simulink model "problem2"  (R2020b)
settings: Solver=VariableStepAuto  StartTime=0.0  StopTime=10.0  RelTol=1e-3
values from neighbouring files (symbols this model uses):
  be = 2.0    [prob2datadic.sldd]
  bv = 1.0    [prob2datadic.sldd]
  Ie = 1.0    [prob2datadic.sldd]
  Iv = 5.0    [prob2datadic.sldd]
  muk = 1.0    [prob2datadic.sldd]
  mus = 1.5    [prob2datadic.sldd]
  R = 1.0    [prob2datadic.sldd]
settings Model: Creator=Nitin  LastModifiedBy=Nitin

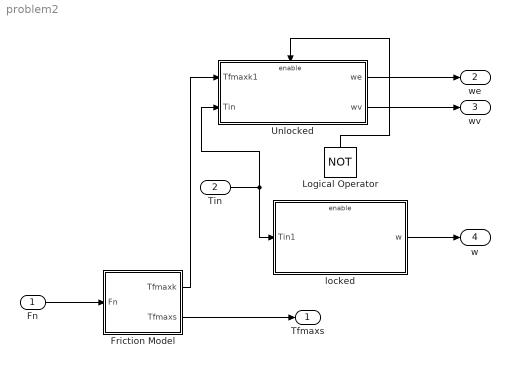
== system problem2 ==
  Fn : Inport
  Tin : Inport  Port=2
  Friction Model : Subsystem
  Logical Operator : Logic  Operator=NOT  OutDataTypeStr=boolean
  Unlocked : Subsystem
  locked : Subsystem
  Tfmaxs : Outport  InitialOutput=0  VectorParamsAs1DForOutWhenUnconnected=off
  we : Outport  Port=2  InitialOutput=0  VectorParamsAs1DForOutWhenUnconnected=off
  wv : Outport  Port=3  InitialOutput=0  VectorParamsAs1DForOutWhenUnconnected=off
  w : Outport  Port=4  InitialOutput=0  VectorParamsAs1DForOutWhenUnconnected=off
  wires:
  Fn/1 -> Friction Model/1(Fn)
  Friction Model/2(Tfmaxs) -> Tfmaxs/1
  Friction Model/1(Tfmaxk) -> Unlocked/1(Tfmaxk1)
  Unlocked/1(we) -> we/1
  Unlocked/2(wv) -> wv/1
  Tin/1 -> Unlocked/2(Tin), locked/1(Tin1)
  locked/1(w) -> w/1
  Logical Operator/1 -> Unlocked/Enable

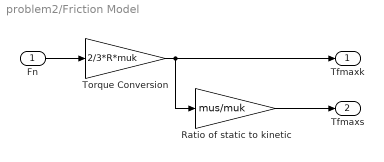
== system problem2/Friction Model ==
  Fn : Inport
  Ratio of static to kinetic : Gain  Gain=mus/muk  SaturateOnIntegerOverflow=on  OutDataTypeStr=Inherit: Same as input  ParamDataTypeStr=Inherit: Same as input
  Torque Conversion : Gain  Gain=2/3*R*muk  SaturateOnIntegerOverflow=on  OutDataTypeStr=Inherit: Same as input  ParamDataTypeStr=Inherit: Same as input
  Tfmaxk : Outport  InitialOutput=0  VectorParamsAs1DForOutWhenUnconnected=off
  Tfmaxs : Outport  Port=2  InitialOutput=0  VectorParamsAs1DForOutWhenUnconnected=off
  wires:
  Fn/1 -> Torque Conversion/1
  Torque Conversion/1 -> Tfmaxk/1, Ratio of static to kinetic/1
  Ratio of static to kinetic/1 -> Tfmaxs/1

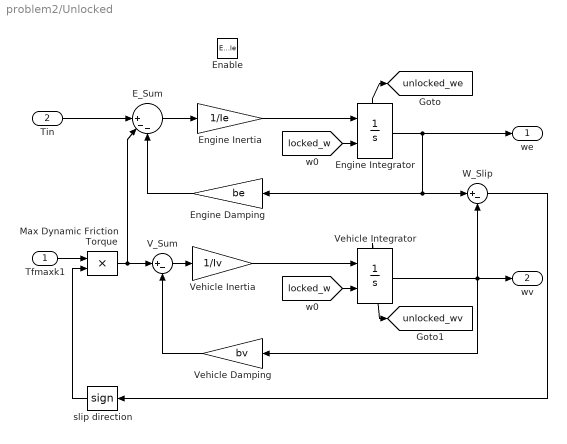
== system problem2/Unlocked ==
  Tfmaxk1 : Inport
  Tin : Inport  Port=2
  Enable : EnablePort  StatesWhenEnabling=reset
  E_Sum : Sum  Inputs=||+--  InputSameDT=on  SaturateOnIntegerOverflow=on  OutDataTypeStr=Inherit: Same as first input
  Engine Damping : Gain  Gain=be  SaturateOnIntegerOverflow=on  OutDataTypeStr=Inherit: Same as input  ParamDataTypeStr=Inherit: Same as input
  Engine Inertia : Gain  Gain=1/Ie  SaturateOnIntegerOverflow=on  OutDataTypeStr=Inherit: Same as input  ParamDataTypeStr=Inherit: Same as input
  Engine Integrator : Integrator  InitialConditionSource=external  ShowStatePort=on
  Max Dynamic Friction Torque : Product  InputSameDT=on  RndMeth=Zero  SaturateOnIntegerOverflow=on  OutDataTypeStr=Inherit: Same as first input
  V_Sum : Sum  Inputs=|+-  InputSameDT=on  SaturateOnIntegerOverflow=on  OutDataTypeStr=Inherit: Same as first input
  Vehicle Damping : Gain  Gain=bv  SaturateOnIntegerOverflow=on  OutDataTypeStr=Inherit: Same as input  ParamDataTypeStr=Inherit: Same as input
  Vehicle Inertia : Gain  Gain=1/Iv  SaturateOnIntegerOverflow=on  OutDataTypeStr=Inherit: Same as input  ParamDataTypeStr=Inherit: Same as input
  Vehicle Integrator : Integrator  InitialConditionSource=external  ShowStatePort=on
  W_Slip : Sum  Inputs=|+-  InputSameDT=on  SaturateOnIntegerOverflow=on  OutDataTypeStr=Inherit: Same as first input
  slip direction : Signum
  we : Outport  InitialOutput=0  VectorParamsAs1DForOutWhenUnconnected=off
  wv : Outport  Port=2  InitialOutput=0  VectorParamsAs1DForOutWhenUnconnected=off
  tag scope: unlocked_we=global, unlocked_wv=global
  wires:
  Engine Integrator/1 -> we/1, Engine Damping/1, W_Slip/1
  Vehicle Integrator/1 -> wv/1, W_Slip/2, Vehicle Damping/1
  Engine Inertia/1 -> Engine Integrator/1
  Engine Damping/1 -> E_Sum/3
  V_Sum/1 -> Vehicle Inertia/1
  Vehicle Inertia/1 -> Vehicle Integrator/1
  [locked_w] -> Engine Integrator/2
  Vehicle Integrator/State -> [unlocked_wv]
  [locked_w] -> Vehicle Integrator/2
  Vehicle Damping/1 -> V_Sum/2
  Tin/1 -> E_Sum/1
  Engine Integrator/State -> [unlocked_we]
  Max Dynamic Friction Torque/1 -> V_Sum/1, E_Sum/2
  Tfmaxk1/1 -> Max Dynamic Friction Torque/1
  E_Sum/1 -> Engine Inertia/1
  slip direction/1 -> Max Dynamic Friction Torque/2
  W_Slip/1 -> slip direction/1

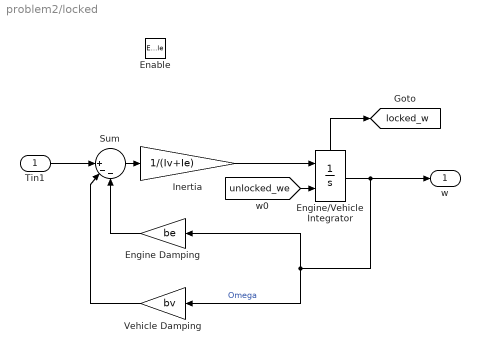
== system problem2/locked ==
  Tin1 : Inport
  Enable : EnablePort  StatesWhenEnabling=reset
  Engine Damping : Gain  Gain=be  SaturateOnIntegerOverflow=on  OutDataTypeStr=Inherit: Same as input  ParamDataTypeStr=Inherit: Same as input
  Engine/Vehicle Integrator : Integrator  InitialConditionSource=external  ShowStatePort=on
  Inertia : Gain  Gain=1/(Iv+Ie)  SaturateOnIntegerOverflow=on  OutDataTypeStr=Inherit: Same as input  ParamDataTypeStr=Inherit: Same as input
  Sum : Sum  Inputs=||+--  InputSameDT=on  SaturateOnIntegerOverflow=on  OutDataTypeStr=Inherit: Same as first input
  Vehicle Damping : Gain  Gain=bv  SaturateOnIntegerOverflow=on  OutDataTypeStr=Inherit: Same as input  ParamDataTypeStr=Inherit: Same as input
  w : Outport  InitialOutput=0  VectorParamsAs1DForOutWhenUnconnected=off
  tag scope: locked_w=global
  wires:
  Sum/1 -> Inertia/1
  [unlocked_we] -> Engine/Vehicle Integrator/2
  Engine/Vehicle Integrator/1 -> w/1, Engine Damping/1, Vehicle Damping/1  "Omega"
  Vehicle Damping/1 -> Sum/2
  Inertia/1 -> Engine/Vehicle Integrator/1
  Engine/Vehicle Integrator/State -> [locked_w]
  Engine Damping/1 -> Sum/3
  Tin1/1 -> Sum/1
